simulink model "mg_simulator"  (Simulink 9.0)
settings: Solver=VariableStepAuto  StartTime=0.0  StopTime=Tsim  FixedStep=.005  MaxStep=Ts  RelTol=1e-6  EnableMultiTasking=on
InitFcn:
  | mg_simulator_init
values from neighbouring files (symbols this model uses):
  B = B + B' + mismatch    [mg_simulator_init.m]    (also in mpc_run_nodewise_mdl_fast.m = B + B'; mpc_run_nodewise_mdl_fast2.m = B + B'; mpc_run_nodewise_mdl_fast3.m = B + B'; mpc_run_nodewise_mdl_fast4.m = B + B')
  g_vector = zeros(1,4)    [mg_simulator_init.m]
  Init = [100; 200; 300; 400]    [mg_simulator_init.m]
  N = 2    [mg_simulator_init.m]
  n_Qi = [1 1 1 1]    [mg_simulator_init.m]
  p_noise = 10*ones(1,4)    [mg_simulator_init.m]
  Q = 10*eye    [mg_simulator_init.m]
  Q_di = 500*ones(1,4)    [mg_simulator_init.m]
  Q_Li = 500*ones(1,4)    [mg_simulator_init.m]
  R = .01*eye    [mg_simulator_init.m]
  tau = 1    [mg_simulator_init.m]
  Thresh = 2    [mg_simulator_init.m]
  Ts = .01    (= 0.01)    [mg_simulator_init.m]
  Ts_noise = .001    (= 0.001)    [mg_simulator_init.m]
  v_ref = 310    [mg_simulator_init.m]
  W = 5*eye    [mg_simulator_init.m]
  w_noise = 1e-3*ones(4,1)'    [mg_simulator_init.m]
  w_noise_est = w_noise    [mg_simulator_init.m]
undefined symbols (not defined in the file or in its folder): magnitude, mpc_run_nodewise_mdl_fast, mpc_run_nodewise_mdl_fast2, mpc_run_nodewise_mdl_fast3
libraries: sharedTrackingLibrary x4
settings Model: SuppressorTable=22 serialization::archive 11 0 6 0 0 0 0 0  Creator=manaswini  LastModifiedBy=seananderson  ExtModeAutoUpdateStatusClock=off
settings DataIOCC: LimitDataPoints=on  SignalLoggingSaveFormat=ModelDataLogs
settings OptimizationCC: ExpressionDepthLimit=2147483647
settings DebuggingCC: AlgebraicLoopMsg=none  SaveWithParameterizedLinksMsg=none  MaxConsecutiveZCsMsg=none  SolverPrmCheckMsg=warning  FcnCallInpInsideContextMsg=warning  StateNameClashWarn=warning
settings HardwareCC: TargetHWDeviceType=32-bit Generic
settings GRTTargetCC: TargetFcnLib=ansi_tfl_tmw.mat  CombineOutputUpdateFcns=off  GRTInterface=on

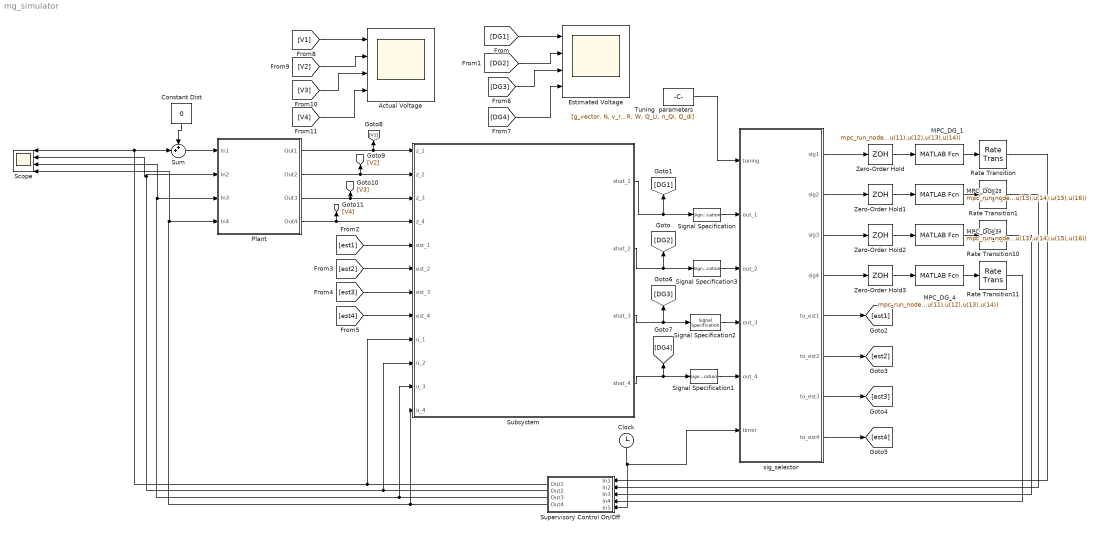
== system mg_simulator ==
  Actual Voltage : Scope  NumInputPorts=4
  Clock : Clock
  Constant Dist : Constant  Value=0
  Estimated Voltage : Scope  NumInputPorts=4
  MPC_DG_1 : MATLABFcn  MATLABFcn=mpc_run_nodewise_mdl_fast(u(1),u(2),u(3),u(4),u(5),u(6),u(7),u(8),u(9),u(10),u(11),u(12),u(13),u(14))  SampleTime=Ts
  MPC_DG_2 : MATLABFcn  MATLABFcn=mpc_run_nodewise_mdl_fast2(u(1),u(2:3),u(4:5),u(6),u(7),u(8),u(9),u(10),u(11),u(12),u(13),u(14),u(15),u(16))  SampleTime=Ts
  MPC_DG_3 : MATLABFcn  MATLABFcn=mpc_run_nodewise_mdl_fast3(u(1),u(2:3),u(4:5),u(6),u(7),u(8),u(9),u(10),u(11),u(12),u(13),u(14),u(15),u(16))  SampleTime=Ts
  MPC_DG_4 : MATLABFcn  MATLABFcn=mpc_run_nodewise_mdl_fast(u(1),u(2),u(3),u(4),u(5),u(6),u(7),u(8),u(9),u(10),u(11),u(12),u(13),u(14))  SampleTime=Ts
  Plant : Subsystem
  Rate Transition{,1,10..11} (4 alike) : RateTransition  OutPortSampleTimeOpt=Inherit  OutPortSampleTime=Ts
  Scope : Scope  NumInputPorts=4
  Signal Specification : SignalSpecification  Dimensions=[ 1 2]
  Signal Specification1 : SignalSpecification  Dimensions=[ 1 2]
  Signal Specification2 : SignalSpecification  Dimensions=[ 1 3]
  Signal Specification3 : SignalSpecification  Dimensions=[ 1 3]
  Subsystem : Subsystem
  Sum : Sum  Inputs=++|
  Supervisory Control On/Off : Subsystem
  Tuning  parameters : Constant  Value=[g_vector, N, v_ref, Ts, Q, R, W, Q_Li, n_Qi, Q_di]
  Zero-Order Hold{,1..3} (4 alike) : ZeroOrderHold  SampleTime=Ts
  sig_selector : MATLAB Function  TreatAsAtomicUnit=on
  wires:
  Clock/1 -> sig_selector/6(timer), Supervisory Control On/Off/5(In5)
  Tuning  parameters/1 -> sig_selector/1(tuning)
  Zero-Order Hold/1 -> MPC_DG_1/1
  sig_selector/1(sig1) -> Zero-Order Hold/1
  MPC_DG_1/1 -> Rate Transition/1
  Rate Transition/1 -> Supervisory Control On/Off/1(In1)
  MPC_DG_2/1 -> Rate Transition1/1
  sig_selector/2(sig2) -> Zero-Order Hold1/1
  Rate Transition1/1 -> Supervisory Control On/Off/2(In2)
  [DG1] -> Estimated Voltage/1
  [DG2] -> Estimated Voltage/2
  sig_selector/5(to_est1) -> [est1]
  sig_selector/6(to_est2) -> [est2]
  Zero-Order Hold1/1 -> MPC_DG_2/1
  Supervisory Control On/Off/1(Out1) -> Subsystem/9(u_1), Sum/2, Scope/1
  Supervisory Control On/Off/2(Out2) -> Subsystem/10(u_2), Scope/2, Plant/2(In2)
  Zero-Order Hold2/1 -> MPC_DG_3/1
  sig_selector/3(sig3) -> Zero-Order Hold2/1
  MPC_DG_3/1 -> Rate Transition10/1
  Zero-Order Hold3/1 -> MPC_DG_4/1
  sig_selector/4(sig4) -> Zero-Order Hold3/1
  MPC_DG_4/1 -> Rate Transition11/1
  sig_selector/7(to_est3) -> [est3]
  sig_selector/8(to_est4) -> [est4]
  Rate Transition10/1 -> Supervisory Control On/Off/3(In3)
  Rate Transition11/1 -> Supervisory Control On/Off/4(In4)
  Supervisory Control On/Off/3(Out3) -> Subsystem/11(u_3), Scope/3, Plant/3(In3)
  Supervisory Control On/Off/4(Out4) -> Subsystem/12(u_4), Scope/4, Plant/4(In4)
  Subsystem/2(xhat_2) -> Signal Specification3/1, [DG2]
  Plant/1(Out1) -> [V1], Subsystem/1(z_1)
  Plant/3(Out3) -> [V3], Subsystem/3(z_3)
  Plant/4(Out4) -> [V4], Subsystem/4(z_4)
  [est1] -> Subsystem/5(est_1)
  [est2] -> Subsystem/6(est_2)
  [est3] -> Subsystem/7(est_3)
  [est4] -> Subsystem/8(est_4)
  Subsystem/4(xhat_4) -> Signal Specification1/1, [DG4]
  Subsystem/3(xhat_3) -> Signal Specification2/1, [DG3]
  [DG3] -> Estimated Voltage/3
  [DG4] -> Estimated Voltage/4
  Signal Specification/1 -> sig_selector/2(out_1)
  Subsystem/1(xhat_1) -> Signal Specification/1, [DG1]
  Signal Specification1/1 -> sig_selector/5(out_4)
  Signal Specification2/1 -> sig_selector/4(out_3)
  Signal Specification3/1 -> sig_selector/3(out_2)
  [V4] -> Actual Voltage/4
  [V3] -> Actual Voltage/3
  [V1] -> Actual Voltage/1
  [V2] -> Actual Voltage/2
  Plant/2(Out2) -> [V2], Subsystem/2(z_2)
  Sum/1 -> Plant/1(In1)
  Constant Dist/1 -> Sum/1

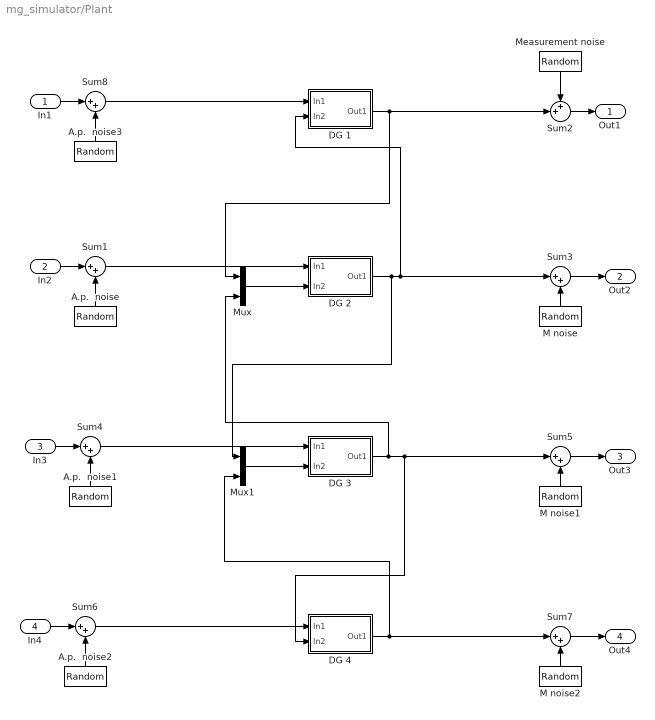
== system mg_simulator/Plant ==
  In1 : Inport
  In2 : Inport  Port=2
  In3 : Inport  Port=3
  In4 : Inport  Port=4
  A.p.  noise : RandomNumber  Variance=p_noise(2)  SampleTime=Ts_noise
  A.p.  noise1 : RandomNumber  Variance=p_noise(2)  SampleTime=Ts_noise
  A.p.  noise2 : RandomNumber  Variance=p_noise(2)  SampleTime=Ts_noise
  A.p.  noise3 : RandomNumber  Variance=p_noise(1)  SampleTime=Ts_noise
  DG 1 : Subsystem  mask{i=1, j=2}
      mask prompts: i "Self ID"; j "Neighbor ID"
  DG 2 : Subsystem  mask{i=2, j1=1, j2=3}
      mask prompts: i "Self ID"; j1 "Neighbor ID"; j2 "Neighbor ID"
  DG 3 : Subsystem  mask{i=3, j1=2, j2=4}
      mask prompts: i "Self ID"; j1 "Neighbor ID"; j2 "Neighbor ID"
  DG 4 : Subsystem  mask{i=4, j=3}
      mask prompts: i "Self ID"; j "Neighbor ID"
  M noise : RandomNumber  Variance=w_noise(2)  SampleTime=Ts_noise
  M noise1 : RandomNumber  Variance=w_noise(2)  SampleTime=Ts_noise
  M noise2 : RandomNumber  Variance=w_noise(2)  SampleTime=Ts_noise
  Measurement noise : RandomNumber  Variance=w_noise(2)  SampleTime=Ts_noise
  Mux : Mux  Inputs=2
  Mux1 : Mux  Inputs=2
  Sum{1,3..8} (7 alike) : Sum  Inputs=|++
  Sum2 : Sum  Inputs=++|
  Out1 : Outport
  Out2 : Outport  Port=2
  Out3 : Outport  Port=3
  Out4 : Outport  Port=4
  wires:
  DG 1/1(Out1) -> Mux/1, Sum2/2
  Sum1/1 -> DG 2/1(In1)
  Sum3/1 -> Out2/1
  M noise/1 -> Sum3/2
  Sum2/1 -> Out1/1
  Measurement noise/1 -> Sum2/1
  In2/1 -> Sum1/1
  A.p.  noise/1 -> Sum1/2
  Sum4/1 -> DG 3/1(In1)
  DG 3/1(Out1) -> Mux/2, DG 4/2(In2), Sum5/1
  DG 2/1(Out1) -> Mux1/1, Sum3/1, DG 1/2(In2)
  A.p.  noise1/1 -> Sum4/2
  Sum5/1 -> Out3/1
  M noise1/1 -> Sum5/2
  In3/1 -> Sum4/1
  Sum6/1 -> DG 4/1(In1)
  DG 4/1(Out1) -> Mux1/2, Sum7/1
  A.p.  noise2/1 -> Sum6/2
  Sum7/1 -> Out4/1
  M noise2/1 -> Sum7/2
  In4/1 -> Sum6/1
  Mux/1 -> DG 2/2(In2)
  Mux1/1 -> DG 3/2(In2)
  In1/1 -> Sum8/1
  A.p.  noise3/1 -> Sum8/2
  Sum8/1 -> DG 1/1(In1)

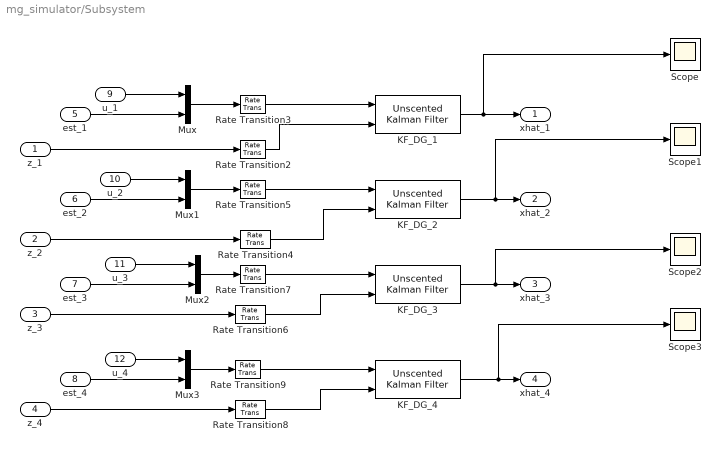
== system mg_simulator/Subsystem ==
  z_1 : Inport
  z_2 : Inport  Port=2
  z_3 : Inport  Port=3
  z_4 : Inport  Port=4
  est_1 : Inport  Port=5
  est_2 : Inport  Port=6
  est_3 : Inport  Port=7
  est_4 : Inport  Port=8
  u_1 : Inport  Port=9
  u_2 : Inport  Port=10
  u_3 : Inport  Port=11
  u_4 : Inport  Port=12
  KF_DG_1 : sharedTrackingLibrary/Unscented Kalman Filter  StateTransitionFcn=estimator_pflow_dynamics  HasAdditiveProcessNoise=Nonadditive  ProcessNoise=p_noise_est{i}  HasTimeVaryingProcessNoise=off  HasStateTransitionFcnExtraArgument=1  InitialState=init_state{i}  InitialStateCovariance=p_noise_est{i}  Alpha=1e-1  Beta=2  Kappa=0  MeasurementFcn1=estimator_measurementFcn  HasMeasurementEnablePort1=off  HasAdditiveMeasurementNoise1=Nonadditive  MeasurementNoise1=w_noise_est(i)  HasTimeVaryingMeasurementNoise1=off  HasMeasurementFcnExtraArgument1=0  MeasurementFcn2=myMeasurementFcn  HasMeasurementEnablePort2=off  HasAdditiveMeasurementNoise2=Additive  MeasurementNoise2=1  HasTimeVaryingMeasurementNoise2=off  HasMeasurementFcnExtraArgument2=0  MeasurementFcn3=myMeasurementFcn  HasMeasurementEnablePort3=off  HasAdditiveMeasurementNoise3=Additive  MeasurementNoise3=1  HasTimeVaryingMeasurementNoise3=off  HasMeasurementFcnExtraArgument3=0  MeasurementFcn4=myMeasurementFcn  HasMeasurementEnablePort4=off  HasAdditiveMeasurementNoise4=Additive  MeasurementNoise4=1  HasTimeVaryingMeasurementNoise4=off  HasMeasurementFcnExtraArgument4=0  MeasurementFcn5=myMeasurementFcn  HasMeasurementEnablePort5=off  HasAdditiveMeasurementNoise5=Additive  MeasurementNoise5=1  HasTimeVaryingMeasurementNoise5=off  HasMeasurementFcnExtraArgument5=0  EnableMultirate=off  StateTransitionFcnSampleTime=1  MeasurementFcn1SampleTime=1  MeasurementFcn2SampleTime=1  MeasurementFcn3SampleTime=1  MeasurementFcn4SampleTime=1  MeasurementFcn5SampleTime=1  UseCurrentEstimator=on  OutputStateCovariance=off  DataType=double  SampleTime=Ts  NumberOfMeasurements=1  mask(Unscented Kalman Filter){i=1}
      settings: SourceProductName=Control System Toolbox  SourceProductBaseCode=CT
  KF_DG_2 : sharedTrackingLibrary/Unscented Kalman Filter  StateTransitionFcn=estimator_pflow_dynamics2  HasAdditiveProcessNoise=Nonadditive  ProcessNoise=p_noise_est{i}  HasTimeVaryingProcessNoise=off  HasStateTransitionFcnExtraArgument=1  InitialState=init_state{i}  InitialStateCovariance=p_noise_est{i}  Alpha=1e-1  Beta=2  Kappa=0  MeasurementFcn1=estimator_measurementFcn  HasMeasurementEnablePort1=off  HasAdditiveMeasurementNoise1=Nonadditive  MeasurementNoise1=w_noise_est(i)  HasTimeVaryingMeasurementNoise1=off  HasMeasurementFcnExtraArgument1=0  MeasurementFcn2=myMeasurementFcn  HasMeasurementEnablePort2=off  HasAdditiveMeasurementNoise2=Additive  MeasurementNoise2=1  HasTimeVaryingMeasurementNoise2=off  HasMeasurementFcnExtraArgument2=0  MeasurementFcn3=myMeasurementFcn  HasMeasurementEnablePort3=off  HasAdditiveMeasurementNoise3=Additive  MeasurementNoise3=1  HasTimeVaryingMeasurementNoise3=off  HasMeasurementFcnExtraArgument3=0  MeasurementFcn4=myMeasurementFcn  HasMeasurementEnablePort4=off  HasAdditiveMeasurementNoise4=Additive  MeasurementNoise4=1  HasTimeVaryingMeasurementNoise4=off  HasMeasurementFcnExtraArgument4=0  MeasurementFcn5=myMeasurementFcn  HasMeasurementEnablePort5=off  HasAdditiveMeasurementNoise5=Additive  MeasurementNoise5=1  HasTimeVaryingMeasurementNoise5=off  HasMeasurementFcnExtraArgument5=0  EnableMultirate=off  StateTransitionFcnSampleTime=1  MeasurementFcn1SampleTime=1  MeasurementFcn2SampleTime=1  MeasurementFcn3SampleTime=1  MeasurementFcn4SampleTime=1  MeasurementFcn5SampleTime=1  UseCurrentEstimator=on  OutputStateCovariance=off  DataType=double  SampleTime=Ts  NumberOfMeasurements=1  mask(Unscented Kalman Filter){i=2}
      settings: SourceProductName=Control System Toolbox  SourceProductBaseCode=CT
  KF_DG_3 : sharedTrackingLibrary/Unscented Kalman Filter  StateTransitionFcn=estimator_pflow_dynamics2  HasAdditiveProcessNoise=Nonadditive  ProcessNoise=p_noise_est{i}  HasTimeVaryingProcessNoise=off  HasStateTransitionFcnExtraArgument=1  InitialState=init_state{i}  InitialStateCovariance=p_noise_est{i}  Alpha=1e-1  Beta=2  Kappa=0  MeasurementFcn1=estimator_measurementFcn  HasMeasurementEnablePort1=off  HasAdditiveMeasurementNoise1=Nonadditive  MeasurementNoise1=w_noise_est(i)  HasTimeVaryingMeasurementNoise1=off  HasMeasurementFcnExtraArgument1=0  MeasurementFcn2=myMeasurementFcn  HasMeasurementEnablePort2=off  HasAdditiveMeasurementNoise2=Additive  MeasurementNoise2=1  HasTimeVaryingMeasurementNoise2=off  HasMeasurementFcnExtraArgument2=0  MeasurementFcn3=myMeasurementFcn  HasMeasurementEnablePort3=off  HasAdditiveMeasurementNoise3=Additive  MeasurementNoise3=1  HasTimeVaryingMeasurementNoise3=off  HasMeasurementFcnExtraArgument3=0  MeasurementFcn4=myMeasurementFcn  HasMeasurementEnablePort4=off  HasAdditiveMeasurementNoise4=Additive  MeasurementNoise4=1  HasTimeVaryingMeasurementNoise4=off  HasMeasurementFcnExtraArgument4=0  MeasurementFcn5=myMeasurementFcn  HasMeasurementEnablePort5=off  HasAdditiveMeasurementNoise5=Additive  MeasurementNoise5=1  HasTimeVaryingMeasurementNoise5=off  HasMeasurementFcnExtraArgument5=0  EnableMultirate=off  StateTransitionFcnSampleTime=1  MeasurementFcn1SampleTime=1  MeasurementFcn2SampleTime=1  MeasurementFcn3SampleTime=1  MeasurementFcn4SampleTime=1  MeasurementFcn5SampleTime=1  UseCurrentEstimator=on  OutputStateCovariance=off  DataType=double  SampleTime=Ts  NumberOfMeasurements=1  mask(Unscented Kalman Filter){i=3}
      settings: SourceProductName=Control System Toolbox  SourceProductBaseCode=CT
  KF_DG_4 : sharedTrackingLibrary/Unscented Kalman Filter  StateTransitionFcn=estimator_pflow_dynamics  HasAdditiveProcessNoise=Nonadditive  ProcessNoise=p_noise_est{i}  HasTimeVaryingProcessNoise=off  HasStateTransitionFcnExtraArgument=1  InitialState=init_state{i}  InitialStateCovariance=p_noise_est{i}  Alpha=1e-1  Beta=2  Kappa=0  MeasurementFcn1=estimator_measurementFcn  HasMeasurementEnablePort1=off  HasAdditiveMeasurementNoise1=Nonadditive  MeasurementNoise1=w_noise_est(i)  HasTimeVaryingMeasurementNoise1=off  HasMeasurementFcnExtraArgument1=0  MeasurementFcn2=myMeasurementFcn  HasMeasurementEnablePort2=off  HasAdditiveMeasurementNoise2=Additive  MeasurementNoise2=1  HasTimeVaryingMeasurementNoise2=off  HasMeasurementFcnExtraArgument2=0  MeasurementFcn3=myMeasurementFcn  HasMeasurementEnablePort3=off  HasAdditiveMeasurementNoise3=Additive  MeasurementNoise3=1  HasTimeVaryingMeasurementNoise3=off  HasMeasurementFcnExtraArgument3=0  MeasurementFcn4=myMeasurementFcn  HasMeasurementEnablePort4=off  HasAdditiveMeasurementNoise4=Additive  MeasurementNoise4=1  HasTimeVaryingMeasurementNoise4=off  HasMeasurementFcnExtraArgument4=0  MeasurementFcn5=myMeasurementFcn  HasMeasurementEnablePort5=off  HasAdditiveMeasurementNoise5=Additive  MeasurementNoise5=1  HasTimeVaryingMeasurementNoise5=off  HasMeasurementFcnExtraArgument5=0  EnableMultirate=off  StateTransitionFcnSampleTime=1  MeasurementFcn1SampleTime=1  MeasurementFcn2SampleTime=1  MeasurementFcn3SampleTime=1  MeasurementFcn4SampleTime=1  MeasurementFcn5SampleTime=1  UseCurrentEstimator=on  OutputStateCovariance=off  DataType=double  SampleTime=Ts  NumberOfMeasurements=1  mask(Unscented Kalman Filter){i=4}
      settings: SourceProductName=Control System Toolbox  SourceProductBaseCode=CT
  Mux{,1..3} (4 alike) : Mux  Inputs=2
  Rate Transition{2..9} (8 alike) : RateTransition
  Scope{,1..3} (4 alike) : Scope
  xhat_1 : Outport
  xhat_2 : Outport  Port=2
  xhat_3 : Outport  Port=3
  xhat_4 : Outport  Port=4
  wires:
  KF_DG_4/1 -> Scope3/1, xhat_4/1
  Rate Transition2/1 -> KF_DG_1/2
  Mux1/1 -> Rate Transition5/1
  est_1/1 -> Mux/2
  z_1/1 -> Rate Transition2/1
  z_2/1 -> Rate Transition4/1
  Rate Transition4/1 -> KF_DG_2/2
  est_2/1 -> Mux1/2
  KF_DG_2/1 -> Scope1/1, xhat_2/1
  Mux/1 -> Rate Transition3/1
  u_3/1 -> Mux2/1
  est_4/1 -> Mux3/2
  KF_DG_1/1 -> Scope/1, xhat_1/1
  z_4/1 -> Rate Transition8/1
  KF_DG_3/1 -> Scope2/1, xhat_3/1
  z_3/1 -> Rate Transition6/1
  Rate Transition6/1 -> KF_DG_3/2
  Mux2/1 -> Rate Transition7/1
  est_3/1 -> Mux2/2
  Rate Transition8/1 -> KF_DG_4/2
  Mux3/1 -> Rate Transition9/1
  u_4/1 -> Mux3/1
  u_2/1 -> Mux1/1
  u_1/1 -> Mux/1
  Rate Transition3/1 -> KF_DG_1/1
  Rate Transition5/1 -> KF_DG_2/1
  Rate Transition7/1 -> KF_DG_3/1
  Rate Transition9/1 -> KF_DG_4/1

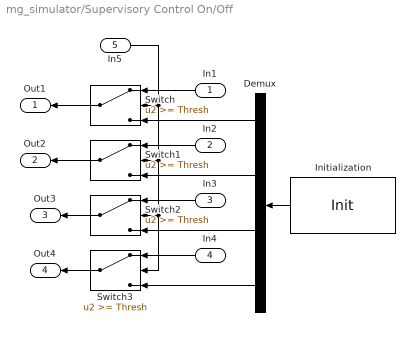
== system mg_simulator/Supervisory Control On/Off ==
  In1 : Inport
  In2 : Inport  Port=2
  In3 : Inport  Port=3
  In4 : Inport  Port=4
  In5 : Inport  Port=5
  Demux : Demux
  Initialization : Constant  Value=Init
  Switch{,1..3} (4 alike) : Switch  Threshold=Thresh
  Out1 : Outport
  Out2 : Outport  Port=2
  Out3 : Outport  Port=3
  Out4 : Outport  Port=4
  wires:
  Demux/2 -> Switch1/3
  Demux/1 -> Switch/3
  Initialization/1 -> Demux/1
  Switch/1 -> Out1/1
  In2/1 -> Switch1/1
  Switch1/1 -> Out2/1
  In5/1 -> Switch3/2, Switch2/2, Switch1/2, Switch/2
  In1/1 -> Switch/1
  Demux/3 -> Switch2/3
  Demux/4 -> Switch3/3
  In3/1 -> Switch2/1
  In4/1 -> Switch3/1
  Switch2/1 -> Out3/1
  Switch3/1 -> Out4/1

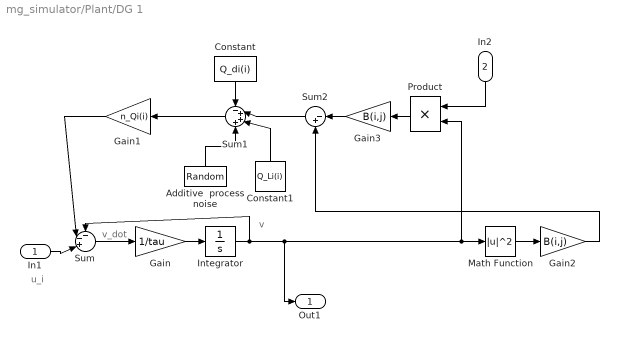
== system mg_simulator/Plant/DG 1 ==
  note: v
  note: v_dot
  note: u_i
  In1 : Inport
  In2 : Inport  Port=2
  Additive  process noise : RandomNumber  Variance=p_noise(i)  SampleTime=Ts_noise  mask{i=1}
  Constant : Constant  Value=Q_di(i)
  Constant1 : Constant  Value=Q_Li(i)
  Gain : Gain  Gain=1/tau
  Gain1 : Gain  Gain=n_Qi(i)
  Gain2 : Gain  Gain=B(i,j)
  Gain3 : Gain  Gain=B(i,j)
  Integrator : Integrator  InitialCondition=Init(1)
  Math Function : Math  Operator=magnitude^2  SaturateOnIntegerOverflow=on
  Product : Product
  Sum : Sum  Inputs=--+|
  Sum1 : Sum  Inputs=-+++
  Sum2 : Sum  Inputs=|-+
  Out1 : Outport
  wires:
  Sum/1 -> Gain/1
  Gain/1 -> Integrator/1
  Integrator/1 -> Math Function/1, Product/2, Out1/1, Sum/1
  In1/1 -> Sum/3
  Gain1/1 -> Sum/2
  Math Function/1 -> Gain2/1
  Sum1/1 -> Gain1/1
  Constant/1 -> Sum1/1
  In2/1 -> Product/1
  Product/1 -> Gain3/1
  Gain3/1 -> Sum2/1
  Gain2/1 -> Sum2/2
  Sum2/1 -> Sum1/2
  Constant1/1 -> Sum1/3
  Additive  process noise/1 -> Sum1/4

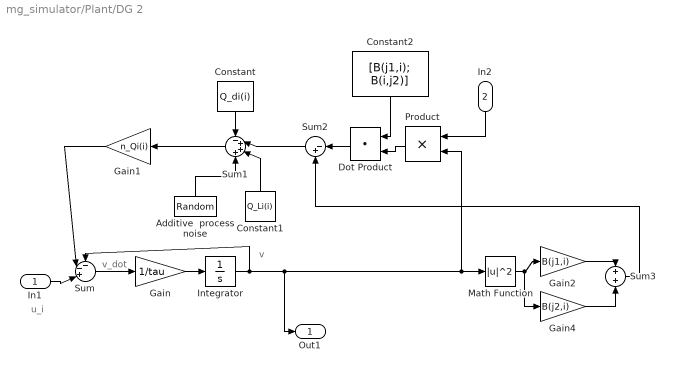
== system mg_simulator/Plant/DG 2 ==
  note: v_dot
  note: u_i
  note: v
  In1 : Inport
  In2 : Inport  Port=2
  Additive  process noise : RandomNumber  Variance=p_noise(i)  SampleTime=Ts_noise  mask{i=2}
  Constant : Constant  Value=Q_di(i)
  Constant1 : Constant  Value=Q_Li(i)
  Constant2 : Constant  Value=[B(j1,i); B(i,j2)]
  Dot Product : DotProduct  InputSameDT=on  OutDataTypeStr=Inherit: Inherit via internal rule
  Gain : Gain  Gain=1/tau
  Gain1 : Gain  Gain=n_Qi(i)
  Gain2 : Gain  Gain=B(j1,i)
  Gain4 : Gain  Gain=B(j2,i)
  Integrator : Integrator  InitialCondition=Init(2)
  Math Function : Math  Operator=magnitude^2  SaturateOnIntegerOverflow=on
  Product : Product
  Sum : Sum  Inputs=--+|
  Sum1 : Sum  Inputs=-+++
  Sum2 : Sum  Inputs=|-+
  Sum3 : Sum
  Out1 : Outport
  wires:
  Gain/1 -> Integrator/1
  Dot Product/1 -> Sum2/1
  In1/1 -> Sum/3
  Math Function/1 -> Gain4/1, Gain2/1
  Sum2/1 -> Sum1/2
  In2/1 -> Product/1
  Gain1/1 -> Sum/2
  Sum/1 -> Gain/1
  Constant/1 -> Sum1/1
  Integrator/1 -> Math Function/1, Product/2, Out1/1, Sum/1
  Constant1/1 -> Sum1/3
  Sum1/1 -> Gain1/1
  Gain2/1 -> Sum3/1
  Gain4/1 -> Sum3/2
  Sum3/1 -> Sum2/2
  Constant2/1 -> Dot Product/1
  Product/1 -> Dot Product/2
  Additive  process noise/1 -> Sum1/4

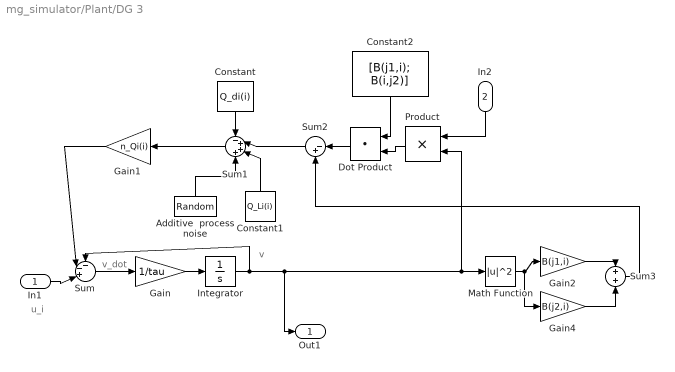
== system mg_simulator/Plant/DG 3 ==
  note: v_dot
  note: u_i
  note: v
  In1 : Inport
  In2 : Inport  Port=2
  Additive  process noise : RandomNumber  Variance=p_noise(i)  SampleTime=Ts_noise  mask{i=2}
  Constant : Constant  Value=Q_di(i)
  Constant1 : Constant  Value=Q_Li(i)
  Constant2 : Constant  Value=[B(j1,i); B(i,j2)]
  Dot Product : DotProduct  InputSameDT=on  OutDataTypeStr=Inherit: Inherit via internal rule
  Gain : Gain  Gain=1/tau
  Gain1 : Gain  Gain=n_Qi(i)
  Gain2 : Gain  Gain=B(j1,i)
  Gain4 : Gain  Gain=B(j2,i)
  Integrator : Integrator  InitialCondition=Init(2)
  Math Function : Math  Operator=magnitude^2  SaturateOnIntegerOverflow=on
  Product : Product
  Sum : Sum  Inputs=--+|
  Sum1 : Sum  Inputs=-+++
  Sum2 : Sum  Inputs=|-+
  Sum3 : Sum
  Out1 : Outport
  wires:
  Gain/1 -> Integrator/1
  Dot Product/1 -> Sum2/1
  In1/1 -> Sum/3
  Math Function/1 -> Gain4/1, Gain2/1
  Sum2/1 -> Sum1/2
  In2/1 -> Product/1
  Gain1/1 -> Sum/2
  Sum/1 -> Gain/1
  Constant/1 -> Sum1/1
  Integrator/1 -> Math Function/1, Product/2, Out1/1, Sum/1
  Constant1/1 -> Sum1/3
  Sum1/1 -> Gain1/1
  Gain2/1 -> Sum3/1
  Gain4/1 -> Sum3/2
  Sum3/1 -> Sum2/2
  Constant2/1 -> Dot Product/1
  Product/1 -> Dot Product/2
  Additive  process noise/1 -> Sum1/4

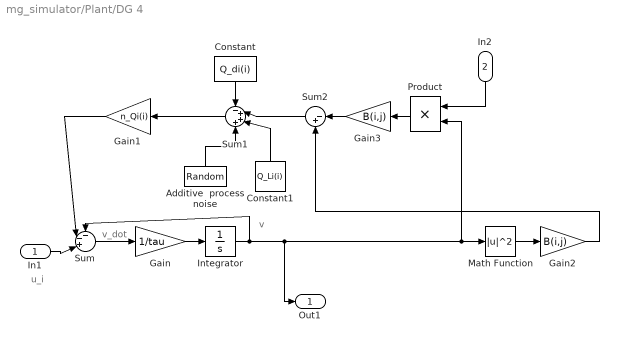
== system mg_simulator/Plant/DG 4 ==
  note: v
  note: v_dot
  note: u_i
  In1 : Inport
  In2 : Inport  Port=2
  Additive  process noise : RandomNumber  Variance=p_noise(i)  SampleTime=Ts_noise  mask{i=1}
  Constant : Constant  Value=Q_di(i)
  Constant1 : Constant  Value=Q_Li(i)
  Gain : Gain  Gain=1/tau
  Gain1 : Gain  Gain=n_Qi(i)
  Gain2 : Gain  Gain=B(i,j)
  Gain3 : Gain  Gain=B(i,j)
  Integrator : Integrator  InitialCondition=Init(1)
  Math Function : Math  Operator=magnitude^2  SaturateOnIntegerOverflow=on
  Product : Product
  Sum : Sum  Inputs=--+|
  Sum1 : Sum  Inputs=-+++
  Sum2 : Sum  Inputs=|-+
  Out1 : Outport
  wires:
  Sum/1 -> Gain/1
  Gain/1 -> Integrator/1
  Integrator/1 -> Math Function/1, Product/2, Out1/1, Sum/1
  In1/1 -> Sum/3
  Gain1/1 -> Sum/2
  Math Function/1 -> Gain2/1
  Sum1/1 -> Gain1/1
  Constant/1 -> Sum1/1
  In2/1 -> Product/1
  Product/1 -> Gain3/1
  Gain3/1 -> Sum2/1
  Gain2/1 -> Sum2/2
  Sum2/1 -> Sum1/2
  Constant1/1 -> Sum1/3
  Additive  process noise/1 -> Sum1/4

== matlab function sig_selector ==
  data: sig1 output double; tuning input double; out_1 input double; out_2 input double; out_3 input double; out_4 input double; sig2 output double; sig3 output double; sig4 output double; timer input double; to_est1 output double; to_est2 output double; to_est3 output double; to_est4 output double
function [sig1, sig2, sig3, sig4, to_est1, to_est2, to_est3, to_est4] = ...
    selector(tuning, out_1, out_2, out_3, out_4, timer)
% [g_vector, N, v_ref, Ts, Q, R, W, Q_Li, n_Qi, Q_di]
g = tuning(1:4);
N = tuning(5);
v_ref = tuning(6);
Ts = tuning(7);
Q = tuning(8);
R = tuning(9);
W = tuning(10);
Q_L_i = tuning(11:14);
n_Qi = tuning(15:18);
Q_di = tuning(19:22);

% create the signals to send to the distributed MPC algorithms
sig1 = [out_1(1), out_1(2), 2, 1, ...
    N, v_ref(1), n_Qi(1), Q_L_i(1), Q_di(1), Ts, Q, W, R, timer]';
sig2 = [out_2(1), [out_2(2), out_2(3)], [1 3], 2, ...
    N, v_ref, n_Qi(2), Q_L_i(2), Q_di(2), Ts, Q, W, R, timer]';
sig3 = [out_3(1), [out_3(2), out_3(3)], [2 4], 3, ...
    N, v_ref, n_Qi(3), Q_L_i(3), Q_di(3), Ts, Q, W, R, timer]';
sig4 = [out_4(1), out_4(2), 3, 4, ...
    N, v_ref, n_Qi(4), Q_L_i(4), Q_di(4), Ts, Q, W, R, timer]';

% create the signals to send to the estimators
to_est1 = double([n_Qi(1), Q_L_i(1), Q_di(1), 2, 1, Ts]);
to_est2 = double([n_Qi(2), Q_L_i(2), Q_di(2), [1 3], 2, Ts]);
to_est3 = double([n_Qi(3), Q_L_i(3), Q_di(3), [2 4], 3, Ts]);
to_est4 = double([n_Qi(4), Q_L_i(4), Q_di(4), 3, 4, Ts]);
end
